simulink model "MAX31856_model"  (R2024a)
settings: Solver=FixedStepAuto  StartTime=0.0  StopTime=tFinal_s  FixedStep=deltaT_s  RelTol=1e-3  EnableMultiTasking=on
libraries: LumArduinoMAX31856 x1
settings Model: SimulationMode=external  ExtModeTrigDuration=2  Creator=Christopher  LastModifiedBy=chris
settings SolverCC: AlgebraicLoopSolver=TrustRegion  AutoInsertRateTranBlk=on
settings DataIOCC: LimitDataPoints=on  StreamToWorkspace=on  ReturnWorkspaceOutputs=off
settings OptimizationCC: LifeSpan=1  MaxStackSize=64
settings DebuggingCC: UnconnectedInputMsg=warning  UnconnectedOutputMsg=warning  UnconnectedLineMsg=warning  AllowSymbolicDim=off  SFUnexpectedBacktrackingDiag=warning  SFNoUnconditionalDefaultTransitionDiag=warning  SFExecutionAtInitializationDiag=none  ArithmeticOperatorsInVariantConditions=warning
settings HardwareCC: ProdBitPerInt=16  ProdBitPerPointer=16  ProdBitPerSizeT=16  ProdBitPerPtrDiffT=16  ProdLargestAtomicFloat=None  ProdWordSize=8  ProdHWDeviceType=Atmel->AVR
settings ModelReferenceCC: EnableRefExpFcnMdlSchedulingChecks=on  PropagateSignalLabelsOutOfModel=off
settings SFSimCC: SimUseLocalCustomCode=off  CustomCodeUndefinedFunction=UseInterfaceOnly
settings RTWCC: Description=Embedded Coder  SystemTargetFile=ert.tlc  HardwareBoard=Arduino Nano 3.0  TemplateMakefile=ert_default_tmf  RTWVerbose=off  RTWUseLocalCustomCode=off  Toolchain=Arduino AVR  BuildConfiguration=Faster Runs  GPUComputeCapability=3.5
settings CodeAppCC: MangleLength=10  StateflowObjectComments=on
settings ERTTargetCC: MultiwordLength=2048  ERTCustomFileBanners=off  SupportContinuousTime=on  SupportNonInlinedSFcns=on  RemoveResetFunc=off  SupportVariableSizeSignals=on  ModelStepFunctionPrototypeControlCompliant=off  ExtMode=on  ExtModeTransport=3  ExtModeStaticAlloc=on  ExtModeAutomaticAllocSize=off  ExtModeStaticAllocSize=250  ExtModeMexFile=ext_xcp  ExtModeMexArgs='127.0.0.1' 0 17725  ExtModeIntrfLevel=Level2 - Open  ERTSrcFileBannerTemplate=codertarget_code_template.cgt  ERTHdrFileBannerTemplate=codertarget_code_template.cgt  ERTDataSrcFileTemplate=codertarget_code_template.cgt  ERTDataHdrFileTemplate=codertarget_code_template.cgt  ConvertIfToSwitch=off  SuppressUnreachableDefaultCases=off
settings ConfigComp: CovMetricSettings=dw  CovSaveCumulativeToWorkspaceVar=on  CovSaveSingleToWorkspaceVar=on  CovExternalEMLEnable=off

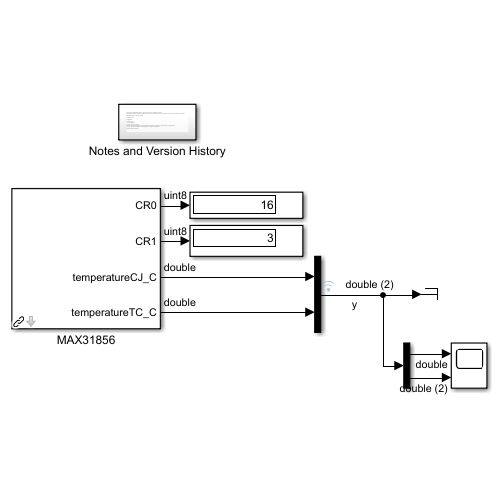
[thumbnail: Simulink's stored preview of the top-level diagram]
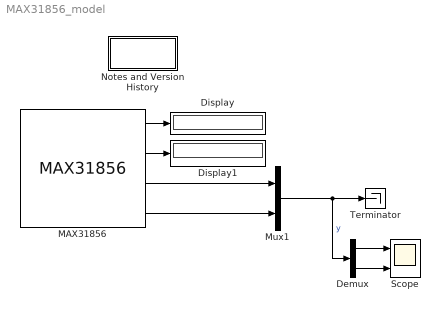
== system MAX31856_model ==
  Demux : Demux  Outputs=2
  Display : Display
  Display1 : Display
  MAX31856 : LumArduinoMAX31856/MAX31856  MAX31856_CR0_REG_READ=MAX31856_CR0_REG_READ  MAX31856_CR0_REG_WRITE=MAX31856_CR0_REG_WRITE  MAX31856_CR1_REG_READ=MAX31856_CR1_REG_READ  MAX31856_CR1_REG_WRITE=MAX31856_CR1_REG_WRITE  MAX31856_MASK_REG_WRITE=MAX31856_MASK_REG_WRITE  MAX31856_CJTO_REG_READ=MAX31856_CJTO_REG_READ  MAX31856_CJTO_REG_WRITE=MAX31856_CJTO_REG_WRITE  MAX31856_CJTH_REG_READ=MAX31856_CJTH_REG_READ  MAX31856_CJTL_REG_READ=MAX31856_CJTL_REG_READ  MAX31856_LTCBH_REG_READ=MAX31856_LTCBH_REG_READ  MAX31856_LTCBM_REG_READ=MAX31856_LTCBM_REG_READ  MAX31856_LTCBL_REG_READ=MAX31856_LTCBL_REG_READ  deltaT_s=deltaT_s  pin_CS=pin_CS
  Mux1 : Mux  Inputs=2
  Notes and Version History : Subsystem
  Scope : Scope  NumInputPorts=2
  Terminator : Terminator
  wires:
  Mux1/1 -> Demux/1, Terminator/1  "y"
  MAX31856/1 -> Display/1
  MAX31856/2 -> Display1/1
  MAX31856/3 -> Mux1/1
  MAX31856/4 -> Mux1/2
  Demux/1 -> Scope/1
  Demux/2 -> Scope/2

== system MAX31856_model/Notes and Version History ==
  note: Interface with a MAX31856 via SPI. This is similar to the functionality outlined in \LumArduinoSDK\Examples\MAX31856\SPI_OneShot\SPI_OneShot.ino except this uses the Simulink Support Package for Arduino Hardware to achieve this functionality.
      |
      | Christopher Lum
      | lum@uw.edu
      |
      | Version History
      | 12/14/24: Created
      | 12/19/24: Continued working
      | 12/20/24: Changed SPI properties via Configuration Parameters > Hardware Implementation > SPI properties
      | 01/04/25: Fixing documentation. Adding support for negative temperatures
      | 01/05/25: Reference library.
